simulink model "uz_pmsm_model_9ph"  (R2021b)
settings: Solver=FixedStepAuto  StartTime=0.0  StopTime=0.8  RelTol=1e-3
PreLoadFcn:
  | uz_pmsm_model_9ph_init_parameter
values from neighbouring files (symbols this model uses):
  c = 2/9*cat(1,tl1,tl2,tl3,tl4,tl5,tl6,tl7,tl8,tl9)    [uz_pmsm_model_9ph_init_parameter.m]
  friction_coefficient = 0.001    [uz_pmsm_model_9ph_init_parameter.m]
  inertia = 0.001    [uz_pmsm_model_9ph_init_parameter.m]
  k_i_d = 50    [uz_pmsm_model_9ph_init_parameter.m]
  k_i_q = 50    [uz_pmsm_model_9ph_init_parameter.m]
  k_p_d = 0.5    [uz_pmsm_model_9ph_init_parameter.m]
  k_p_q = 0.5    [uz_pmsm_model_9ph_init_parameter.m]
  L_d = 0.0023    [uz_pmsm_model_9ph_init_parameter.m]
  L_o1 = L_d/3    (= 0.000766666666667)    [uz_pmsm_model_9ph_init_parameter.m]
  L_o2 = L_d/3    (= 0.000766666666667)    [uz_pmsm_model_9ph_init_parameter.m]
  L_q = 0.0046    [uz_pmsm_model_9ph_init_parameter.m]
  L_x1 = L_d/3    (= 0.000766666666667)    [uz_pmsm_model_9ph_init_parameter.m]
  L_x2 = L_d/3    (= 0.000766666666667)    [uz_pmsm_model_9ph_init_parameter.m]
  L_y1 = L_d/3    (= 0.000766666666667)    [uz_pmsm_model_9ph_init_parameter.m]
  L_y2 = L_d/3    (= 0.000766666666667)    [uz_pmsm_model_9ph_init_parameter.m]
  L_zero = L_d/3    (= 0.000766666666667)    [uz_pmsm_model_9ph_init_parameter.m]
  polepair = 3    [uz_pmsm_model_9ph_init_parameter.m]
  psi_pm = 0.1028    [uz_pmsm_model_9ph_init_parameter.m]
  R_1 = 0.066    [uz_pmsm_model_9ph_init_parameter.m]
  static_friction_torque = 0.001    [uz_pmsm_model_9ph_init_parameter.m]
  ts = 2/1e6    (= 2e-06)    [uz_pmsm_model_9ph_init_parameter.m]
undefined symbols (not defined in the file or in its folder): Kpd, Tnd
libraries: slpidlib x2, simulink x2, spsAlphaBetaZerotodq0Lib x1, pid_lib x1, spsdq0toAlphaBetaZeroLib x1
(part 1 of 2)
settings Model: DataTypeOverride=Off  Creator=ts  LastModifiedBy=ts
settings SolverCC: AlgebraicLoopSolver=TrustRegion  AutoInsertRateTranBlk=on
settings DataIOCC: LimitDataPoints=on  SaveOutput=off  SaveTime=off
settings OptimizationCC: BlockReduction=off  ConditionallyExecuteInputs=off  DefaultParameterBehavior=Inlined  LifeSpan=inf
settings DebuggingCC: AlgebraicLoopMsg=error  SingleTaskRateTransMsg=error  AllowSymbolicDim=off  StrictBusMsg=ErrorOnBusTreatedAsVector  SFUnexpectedBacktrackingDiag=warning  SFNoUnconditionalDefaultTransitionDiag=warning  SFExecutionAtInitializationDiag=none  SFMachineParentedDataDiag=warning  ArithmeticOperatorsInVariantConditions=warning
settings HardwareCC: ProdBitPerPointer=32  ProdBitPerSizeT=32  ProdBitPerPtrDiffT=32  ProdLargestAtomicFloat=None  ProdIntDivRoundTo=Undefined  ProdEndianess=Unspecified  ProdWordSize=32  ProdHWDeviceType=ASIC/FPGA->ASIC/FPGA  ProdEqTarget=off
settings SFSimCC: SimUseLocalCustomCode=off  CustomCodeUndefinedFunction=UseInterfaceOnly
settings RTWCC: RTWUseLocalCustomCode=off
settings CodeAppCC: StateflowObjectComments=on
settings GRTTargetCC: TargetLangStandard=C89/C90 (ANSI)
settings ConfigComp: CovScope=ReferencedModels  CovMetricSettings=dw  CovSaveCumulativeToWorkspaceVar=on  CovSaveSingleToWorkspaceVar=on  CovExternalEMLEnable=off  CovSFcnEnable=off

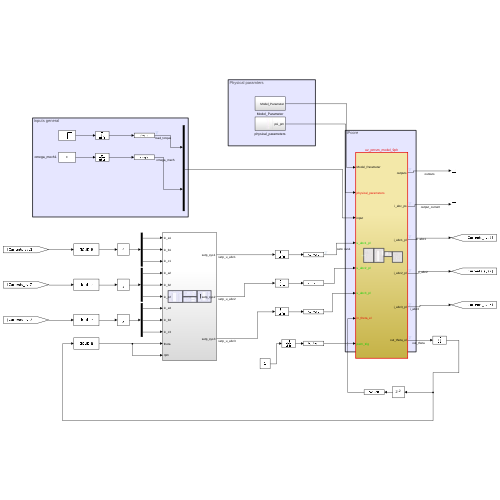
[thumbnail: Simulink's stored preview of the top-level diagram]
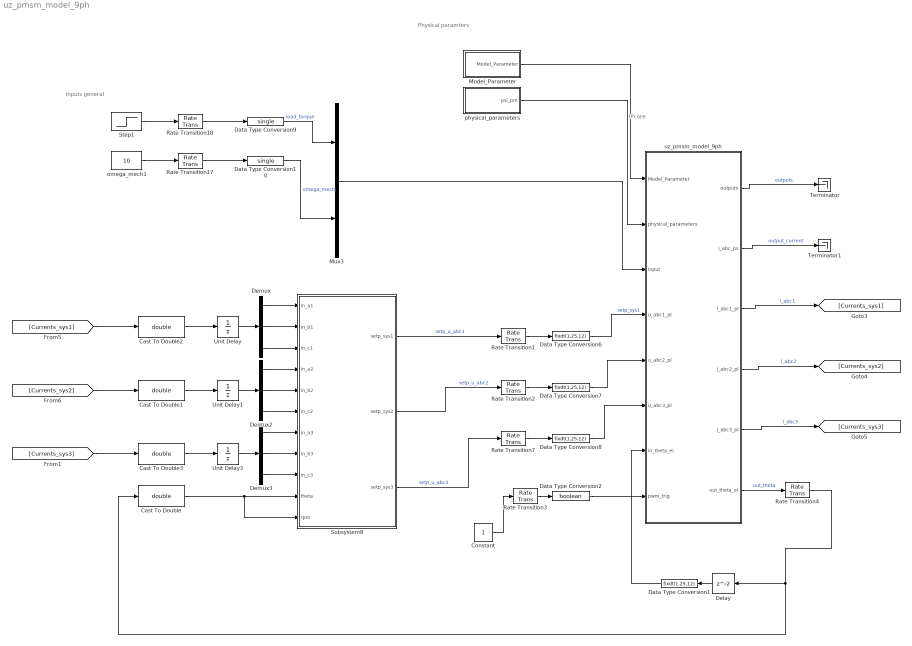
== system uz_pmsm_model_9ph ==
  note: IPcore
  note: Physical paramters
  note: Inputs general
  Cast To Double{,1..3} (4 alike) : DataTypeConversion  OutDataTypeStr=double
  Constant : Constant
  Data Type Conversion{1,6..8} (4 alike) : DataTypeConversion  OutDataTypeStr=fixdt(1,25,12)  RndMeth=Nearest
  Data Type Conversion10 : DataTypeConversion  OutDataTypeStr=single  RndMeth=Nearest
  Data Type Conversion2 : DataTypeConversion  OutDataTypeStr=boolean  RndMeth=Nearest
  Data Type Conversion9 : DataTypeConversion  OutDataTypeStr=single  RndMeth=Nearest
  Delay : Delay
  Demux : Demux  Outputs=3
  Demux2 : Demux  Outputs=3
  Demux3 : Demux  Outputs=3
  Model_Parameter : Subsystem
  Mux3 : Mux  Inputs=2
  Rate Transition{1..4,7,17..18} (7 alike) : RateTransition  OutPortSampleTime=ts
  Step1 : Step  Time=0.25  After=20  SampleTime=0
  Subsystem8 : Subsystem
  Terminator : Terminator
  Terminator1 : Terminator
  Unit Delay : UnitDelay  SampleTime=-1  HasFrameUpgradeWarning=on
  Unit Delay1 : UnitDelay  SampleTime=-1  HasFrameUpgradeWarning=on
  Unit Delay3 : UnitDelay  SampleTime=-1  HasFrameUpgradeWarning=on
  omega_mech1 : Constant  Value=10
  physical_parameters : Subsystem
  uz_pmsm_model_9ph : Subsystem  TreatAsAtomicUnit=on
  wires:
  physical_parameters/1(psi_pm) -> uz_pmsm_model_9ph/2(physical_parameters)
  uz_pmsm_model_9ph/1(outputs) -> Terminator/1  "outputs"
  Model_Parameter/1(Model_Parameter) -> uz_pmsm_model_9ph/1(Model_Parameter)
  omega_mech1/1 -> Rate Transition17/1
  Rate Transition18/1 -> Data Type Conversion9/1
  Step1/1 -> Rate Transition18/1
  Data Type Conversion10/1 -> Mux3/2  "omega_mech"
  Rate Transition17/1 -> Data Type Conversion10/1
  Data Type Conversion9/1 -> Mux3/1  "load_torque"
  Mux3/1 -> uz_pmsm_model_9ph/3(input)
  Data Type Conversion1/1 -> uz_pmsm_model_9ph/7(in_theta_el)
  uz_pmsm_model_9ph/2(i_abc_ps) -> Terminator1/1  "output_current"
  uz_pmsm_model_9ph/3(i_abc1_pl) -> [Currents_sys1]  "i_abc1"
  uz_pmsm_model_9ph/5(i_abc3_pl) -> [Currents_sys3]  "i_abc3"
  uz_pmsm_model_9ph/4(i_abc2_pl) -> [Currents_sys2]  "i_abc2"
  uz_pmsm_model_9ph/6(out_theta_el) -> Rate Transition4/1  "out_theta"
  Delay/1 -> Data Type Conversion1/1
  Subsystem8/1(setp_sys1) -> Rate Transition1/1  "setp_u_abc1"
  Data Type Conversion6/1 -> uz_pmsm_model_9ph/4(u_abc1_pl)  "setp_sys1"
  Subsystem8/2(setp_sys2) -> Rate Transition2/1  "setp_u_abc2"
  Subsystem8/3(setp_sys3) -> Rate Transition7/1  "setp_u_abc3"
  Data Type Conversion8/1 -> uz_pmsm_model_9ph/6(u_abc3_pl)
  Data Type Conversion7/1 -> uz_pmsm_model_9ph/5(u_abc2_pl)
  Unit Delay3/1 -> Demux3/1
  Demux/2 -> Subsystem8/2(in_b1)
  Demux2/1 -> Subsystem8/4(in_a2)
  Demux3/2 -> Subsystem8/8(in_b3)
  Unit Delay1/1 -> Demux2/1
  Demux/3 -> Subsystem8/3(in_c1)
  [Currents_sys1] -> Cast To Double2/1
  [Currents_sys2] -> Cast To Double1/1
  Demux3/3 -> Subsystem8/9(in_c3)
  Unit Delay/1 -> Demux/1
  [Currents_sys3] -> Cast To Double3/1
  Demux3/1 -> Subsystem8/7(in_a3)
  Demux/1 -> Subsystem8/1(in_a1)
  Demux2/2 -> Subsystem8/5(in_b2)
  Demux2/3 -> Subsystem8/6(in_c2)
  Cast To Double/1 -> Subsystem8/11(rpm), Subsystem8/10(theta)
  Cast To Double1/1 -> Unit Delay1/1
  Cast To Double2/1 -> Unit Delay/1
  Cast To Double3/1 -> Unit Delay3/1
  Rate Transition1/1 -> Data Type Conversion6/1
  Rate Transition2/1 -> Data Type Conversion7/1
  Rate Transition7/1 -> Data Type Conversion8/1
  Data Type Conversion2/1 -> uz_pmsm_model_9ph/8(pwm_trig)
  Rate Transition3/1 -> Data Type Conversion2/1
  Constant/1 -> Rate Transition3/1
  Rate Transition4/1 -> Delay/1, Cast To Double/1

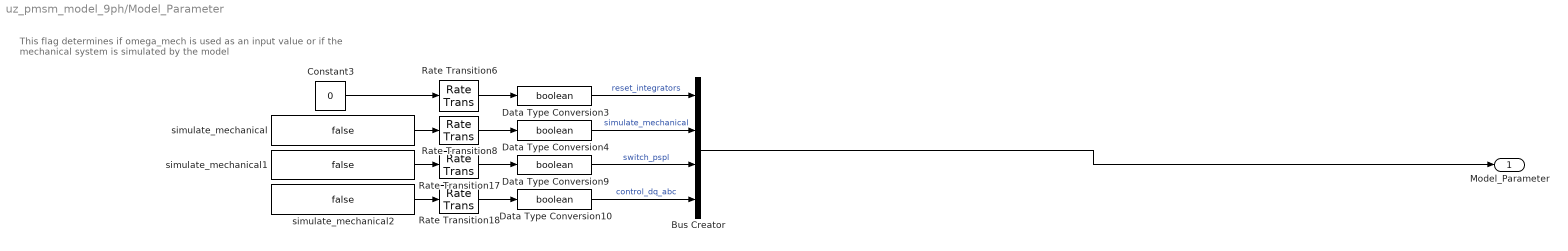
== system uz_pmsm_model_9ph/Model_Parameter ==
  note: This flag determines if omega_mech is used as an input value or
      | if the mechanical system is simulated by the model
  Bus Creator : BusCreator  Inputs=4
  Constant3 : Constant  Value=0
  Data Type Conversion{3..4,9..10} (4 alike) : DataTypeConversion  OutDataTypeStr=boolean
  Rate Transition{6,8,17..18} (4 alike) : RateTransition  OutPortSampleTime=ts
  simulate_mechanical : Constant  Value=false
  simulate_mechanical1 : Constant  Value=false
  simulate_mechanical2 : Constant  Value=false
  Model_Parameter : Outport
  wires:
  simulate_mechanical2/1 -> Rate Transition18/1
  simulate_mechanical/1 -> Rate Transition8/1
  Rate Transition8/1 -> Data Type Conversion4/1
  Rate Transition6/1 -> Data Type Conversion3/1
  Constant3/1 -> Rate Transition6/1
  simulate_mechanical1/1 -> Rate Transition17/1
  Rate Transition17/1 -> Data Type Conversion9/1
  Rate Transition18/1 -> Data Type Conversion10/1
  Data Type Conversion10/1 -> Bus Creator/4  "control_dq_abc"
  Data Type Conversion9/1 -> Bus Creator/3  "switch_pspl"
  Data Type Conversion4/1 -> Bus Creator/2  "simulate_mechanical"
  Bus Creator/1 -> Model_Parameter/1
  Data Type Conversion3/1 -> Bus Creator/1  "reset_integrators"

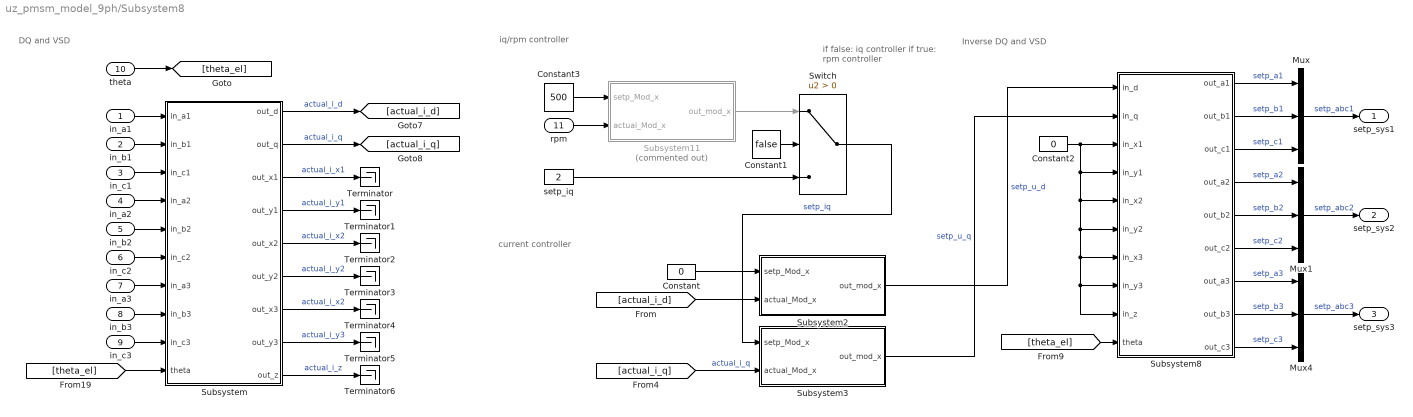
== system uz_pmsm_model_9ph/Subsystem8 ==
  note: DQ and VSD
  note: current controller
  note: iq/rpm controller
  note: if false: iq controller
      | if true: rpm controller
  note: Inverse DQ and VSD
  in_a1 : Inport
  in_b1 : Inport  Port=2
  in_c1 : Inport  Port=3
  in_a2 : Inport  Port=4
  in_b2 : Inport  Port=5
  in_c2 : Inport  Port=6
  in_a3 : Inport  Port=7
  in_b3 : Inport  Port=8
  in_c3 : Inport  Port=9
  theta : Inport  Port=10
  rpm : Inport  Port=11
  Constant : Constant  Value=0
  Constant1 : Constant  Value=false
  Constant2 : Constant  Value=0
  Constant3 : Constant  Value=500
  Mux : Mux  Inputs=3
  Mux1 : Mux  Inputs=3
  Mux4 : Mux  Inputs=3
  Subsystem : Subsystem
  Subsystem11 : Subsystem  Commented=on
  Subsystem2 : Subsystem
  Subsystem3 : Subsystem
  Subsystem8 : Subsystem
  Switch : Switch  Criteria=u2 > Threshold
  Terminator{,1..6} (7 alike) : Terminator
  setp_iq : Constant  Value=2
  setp_sys1 : Outport
  setp_sys2 : Outport  Port=2
  setp_sys3 : Outport  Port=3
  wires:
  Subsystem/4(out_y1) -> Terminator1/1  "actual_i_y1"
  Subsystem8/1(out_a1) -> Mux/1  "setp_a1"
  in_b1/1 -> Subsystem/2(in_b1)
  [theta_el] -> Subsystem8/10(theta)
  Subsystem8/2(out_b1) -> Mux/2  "setp_b1"
  Subsystem8/3(out_c1) -> Mux/3  "setp_c1"
  Subsystem/3(out_x1) -> Terminator/1  "actual_i_x1"
  in_c1/1 -> Subsystem/3(in_c1)
  [actual_i_d] -> Subsystem2/2(actual_Mod_x)
  Constant/1 -> Subsystem2/1(setp_Mod_x)
  Subsystem/6(out_y2) -> Terminator3/1  "actual_i_y2"
  Subsystem/5(out_x2) -> Terminator2/1  "actual_i_x2"
  in_a1/1 -> Subsystem/1(in_a1)
  [actual_i_q] -> Subsystem3/2(actual_Mod_x)  "actual_i_q"
  in_b2/1 -> Subsystem/5(in_b2)
  in_a2/1 -> Subsystem/4(in_a2)
  in_c2/1 -> Subsystem/6(in_c2)
  theta/1 -> [theta_el]
  Mux/1 -> setp_sys1/1  "setp_abc1"
  Subsystem/8(out_y3) -> Terminator5/1  "actual_i_y3"
  Subsystem/7(out_x3) -> Terminator4/1  "actual_i_x2"
  Subsystem/9(out_z) -> Terminator6/1  "actual_i_z"
  in_c3/1 -> Subsystem/9(in_c3)
  in_b3/1 -> Subsystem/8(in_b3)
  in_a3/1 -> Subsystem/7(in_a3)
  Mux1/1 -> setp_sys2/1  "setp_abc2"
  Subsystem8/6(out_c2) -> Mux1/3  "setp_c2"
  Subsystem8/5(out_b2) -> Mux1/2  "setp_b2"
  Subsystem8/4(out_a2) -> Mux1/1  "setp_a2"
  Mux4/1 -> setp_sys3/1  "setp_abc3"
  Subsystem8/7(out_a3) -> Mux4/1  "setp_a3"
  Subsystem8/8(out_b3) -> Mux4/2  "setp_b3"
  Subsystem8/9(out_c3) -> Mux4/3  "setp_c3"
  rpm/1 -> Subsystem11/2(actual_Mod_x)
  Subsystem/1(out_d) -> [actual_i_d]  "actual_i_d"
  Subsystem/2(out_q) -> [actual_i_q]  "actual_i_q"
  [theta_el] -> Subsystem/10(theta)
  Constant2/1 -> Subsystem8/3(in_x1), Subsystem8/8(in_y3), Subsystem8/9(in_z), Subsystem8/7(in_x3), Subsystem8/6(in_y2), Subsystem8/5(in_x2), Subsystem8/4(in_y1)
  Subsystem11/1(out_mod_x) -> Switch/1
  Switch/1 -> Subsystem3/1(setp_Mod_x)  "setp_iq"
  Constant1/1 -> Switch/2
  setp_iq/1 -> Switch/3
  Constant3/1 -> Subsystem11/1(setp_Mod_x)
  Subsystem3/1(out_mod_x) -> Subsystem8/2(in_q)  "setp_u_q"
  Subsystem2/1(out_mod_x) -> Subsystem8/1(in_d)  "setp_u_d"

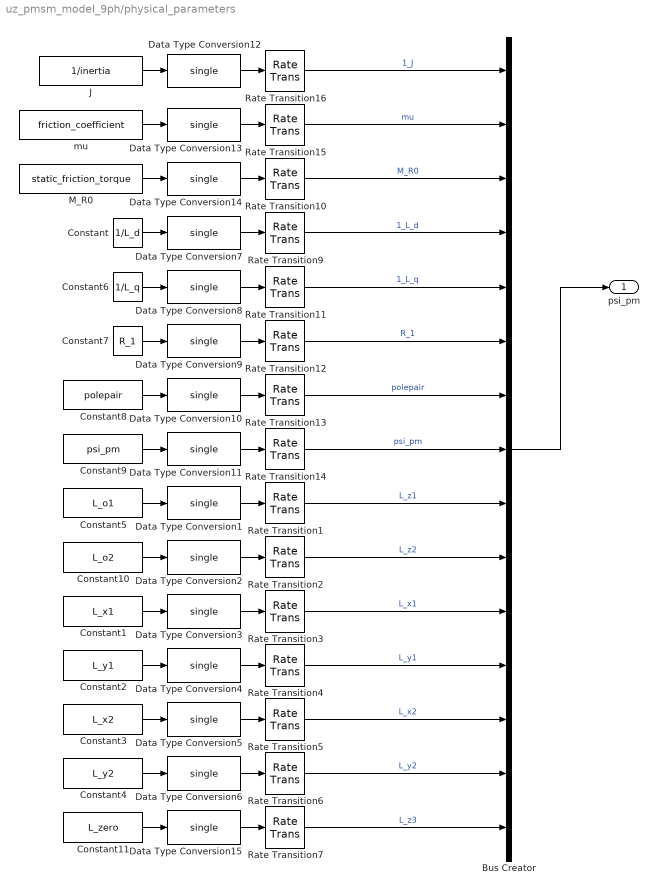
== system uz_pmsm_model_9ph/physical_parameters ==
  Bus Creator : BusCreator  Inputs=15
  Constant : Constant  Value=1/L_d
  Constant1 : Constant  Value=L_x1
  Constant10 : Constant  Value=L_o2
  Constant11 : Constant  Value=L_zero
  Constant2 : Constant  Value=L_y1
  Constant3 : Constant  Value=L_x2
  Constant4 : Constant  Value=L_y2
  Constant5 : Constant  Value=L_o1
  Constant6 : Constant  Value=1/L_q
  Constant7 : Constant  Value=R_1
  Constant8 : Constant  Value=polepair
  Constant9 : Constant  Value=psi_pm
  Data Type Conversion{1..15} (15 alike) : DataTypeConversion  OutDataTypeStr=single
  J : Constant  Value=1/inertia
  M_R0 : Constant  Value=static_friction_torque
  Rate Transition{1..7,9..16} (15 alike) : RateTransition  OutPortSampleTime=ts
  mu : Constant  Value=friction_coefficient
  psi_pm : Outport
  wires:
  Data Type Conversion12/1 -> Rate Transition16/1
  Data Type Conversion7/1 -> Rate Transition9/1
  Rate Transition10/1 -> Bus Creator/3  "M_R0"
  Rate Transition14/1 -> Bus Creator/8  "psi_pm"
  Data Type Conversion14/1 -> Rate Transition10/1
  Rate Transition12/1 -> Bus Creator/6  "R_1"
  Rate Transition16/1 -> Bus Creator/1  "1_J"
  Rate Transition13/1 -> Bus Creator/7  "polepair"
  Bus Creator/1 -> psi_pm/1
  Data Type Conversion11/1 -> Rate Transition14/1
  Constant8/1 -> Data Type Conversion10/1
  Data Type Conversion9/1 -> Rate Transition12/1
  Rate Transition15/1 -> Bus Creator/2  "mu"
  Constant6/1 -> Data Type Conversion8/1
  Rate Transition9/1 -> Bus Creator/4  "1_L_d"
  J/1 -> Data Type Conversion12/1
  Data Type Conversion8/1 -> Rate Transition11/1
  Data Type Conversion10/1 -> Rate Transition13/1
  mu/1 -> Data Type Conversion13/1
  M_R0/1 -> Data Type Conversion14/1
  Rate Transition11/1 -> Bus Creator/5  "1_L_q"
  Data Type Conversion13/1 -> Rate Transition15/1
  Constant7/1 -> Data Type Conversion9/1
  Constant9/1 -> Data Type Conversion11/1
  Constant/1 -> Data Type Conversion7/1
  Data Type Conversion1/1 -> Rate Transition1/1
  Data Type Conversion2/1 -> Rate Transition2/1
  Data Type Conversion3/1 -> Rate Transition3/1
  Data Type Conversion4/1 -> Rate Transition4/1
  Data Type Conversion5/1 -> Rate Transition5/1
  Data Type Conversion6/1 -> Rate Transition6/1
  Constant11/1 -> Data Type Conversion15/1
  Data Type Conversion15/1 -> Rate Transition7/1
  Rate Transition1/1 -> Bus Creator/9  "L_z1"
  Rate Transition7/1 -> Bus Creator/15  "L_z3"
  Rate Transition6/1 -> Bus Creator/14  "L_y2"
  Rate Transition5/1 -> Bus Creator/13  "L_x2"
  Rate Transition4/1 -> Bus Creator/12  "L_y1"
  Rate Transition3/1 -> Bus Creator/11  "L_x1"
  Rate Transition2/1 -> Bus Creator/10  "L_z2"
  Constant4/1 -> Data Type Conversion6/1
  Constant3/1 -> Data Type Conversion5/1
  Constant2/1 -> Data Type Conversion4/1
  Constant1/1 -> Data Type Conversion3/1
  Constant5/1 -> Data Type Conversion1/1
  Constant10/1 -> Data Type Conversion2/1

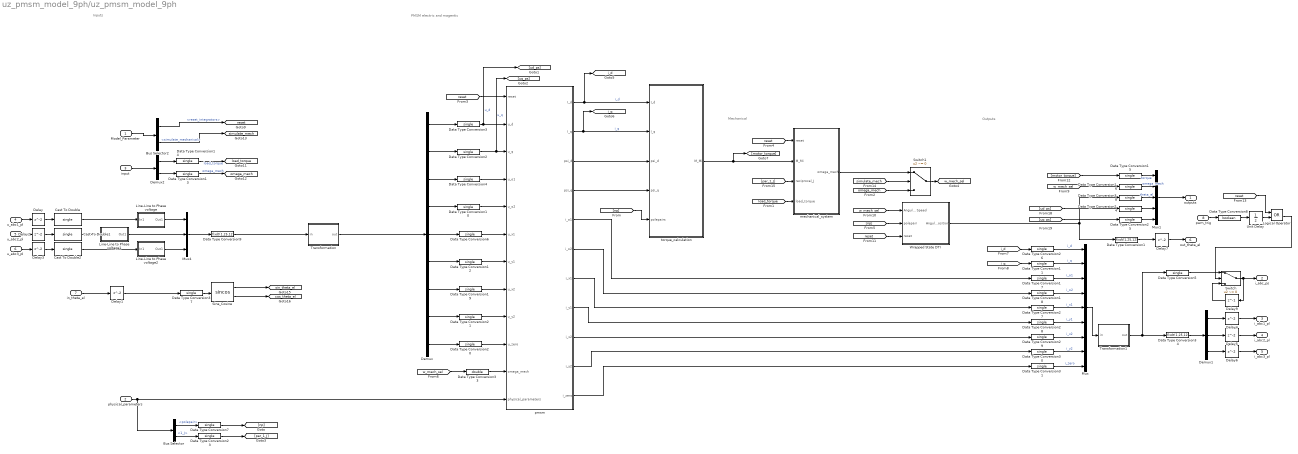
== system uz_pmsm_model_9ph/uz_pmsm_model_9ph ==
  note: PMSM electric and magentic
  note: Mechanical
  note: Outputs
  note: Inputs
  Model_Parameter : Inport
  physical_parameters : Inport  Port=2
  input : Inport  Port=3
  u_abc1_pl : Inport  Port=4
  u_abc2_pl : Inport  Port=5
  u_abc3_pl : Inport  Port=6
  in_theta_el : Inport  Port=7
  pwm_trig : Inport  Port=8
  Bus Selector : BusSelector  OutputSignals=polepair,1_J
  Bus Selector2 : BusSelector  OutputSignals=reset_integrators,simulate_mechanical
  Cast To Double : DataTypeConversion  OutDataTypeStr=single
  Cast To Double1 : DataTypeConversion  OutDataTypeStr=single
  Cast To Double2 : DataTypeConversion  OutDataTypeStr=single
  Data Type Conversion1 : DataTypeConversion  OutDataTypeStr=fixdt(1,25,12)  RndMeth=Nearest
  Data Type Conversion{2..7,10..21,23..31,37..38} (29 alike) : DataTypeConversion  OutDataTypeStr=single  RndMeth=Nearest
  Data Type Conversion33 : DataTypeConversion  OutDataTypeStr=double  RndMeth=Nearest
  Data Type Conversion34 : DataTypeConversion  OutDataTypeStr=fixdt(1,25,12)  RndMeth=Nearest
  Data Type Conversion8 : DataTypeConversion  OutDataTypeStr=boolean  RndMeth=Nearest
  Data Type Conversion9 : DataTypeConversion  OutDataTypeStr=fixdt(1,25,12)  RndMeth=Nearest
  Delay{,1..7} (8 alike) : Delay
  Delay9 : Delay  DelayLength=1
  Demux : Demux  Outputs=9
  Demux1 : Demux  Outputs=3
  Demux2 : Demux  Outputs=2
  Line-Line to Phase voltage : Subsystem
  Line-Line to Phase voltage1 : Subsystem
  Line-Line to Phase voltage2 : Subsystem
  Logical Operator : Logic  Operator=OR  AllPortsSameDT=off  OutDataTypeStr=boolean
  Mux : Mux  Inputs=9
  Mux1 : Mux  Inputs=5
  Mux4 : Mux  Inputs=3
  Sine_Cosine : Trigonometry  Operator=sincos
  Switch : Switch  Criteria=u2 ~= 0
  Switch1 : Switch  Criteria=u2 ~= 0
  Transformation : Subsystem
  Transformation1 : Subsystem
  Unit Delay : UnitDelay  SampleTime=-1  HasFrameUpgradeWarning=on
  Wrapped State DTI : Subsystem
  mechanical_system : Subsystem
  pmsm : Subsystem
  torque_calculation : Subsystem
  outputs : Outport
  i_abc_ps : Outport  Port=2
  i_abc1_pl : Outport  Port=3
  i_abc2_pl : Outport  Port=4
  i_abc3_pl : Outport  Port=5
  out_theta_el : Outport  Port=6
  tag scope: cos_theta_el=global, i_d=global, i_q=global, load_torque=global, omega_mech=global, reset=global, simulate_mech=global, sin_theta_el=global, w_mech_sel=global
  wires:
  pmsm/3(psi_d) -> torque_calculation/3(psi_d)
  pmsm/4(psi_q) -> torque_calculation/4(psi_q)
  Data Type Conversion3/1 -> [ud_ps], pmsm/2(u_d)  "u_d"
  [simulate_mech] -> Switch1/2
  torque_calculation/1(M_Mi) -> [motor_torque], mechanical_system/2(M_Mi)
  physical_parameters/1 -> pmsm/12(physical_parameters), Bus Selector/1
  Data Type Conversion2/1 -> [uq_ps], pmsm/3(u_q)  "u_q"
  mechanical_system/1(omega_mech) -> Switch1/1
  pmsm/2(I_q) -> [i_q], torque_calculation/2(I_q)  "i_q"
  pmsm/1(I_d) -> [i_d], torque_calculation/1(I_d)  "i_d"
  Data Type Conversion16/1 -> Mux1/2  "omega_mech"
  Data Type Conversion15/1 -> Mux1/1  "torque"
  Data Type Conversion11/1 -> Mux/2  "i_q"
  Demux/1 -> Data Type Conversion3/1
  Demux/2 -> Data Type Conversion2/1
  [np] -> torque_calculation/5(polepairs)
  [load_torque] -> mechanical_system/4(load_torque)
  [omega_mech] -> Switch1/3
  Demux/3 -> Data Type Conversion4/1
  Demux/4 -> Data Type Conversion10/1
  Demux/5 -> Data Type Conversion6/1
  Demux/6 -> Data Type Conversion12/1
  Demux/7 -> Data Type Conversion19/1
  Demux/8 -> Data Type Conversion21/1
  Demux/9 -> Data Type Conversion20/1
  Data Type Conversion4/1 -> pmsm/4(u_o1)
  Data Type Conversion10/1 -> pmsm/5(u_o2)
  Data Type Conversion6/1 -> pmsm/6(u_x1)
  Data Type Conversion12/1 -> pmsm/7(u_y1)
  Data Type Conversion19/1 -> pmsm/8(u_x2)
  Data Type Conversion20/1 -> pmsm/10(u_zero)
  Data Type Conversion17/1 -> Mux/3  "i_o1"
  Data Type Conversion18/1 -> Mux/4  "i_o2"
  pmsm/5(i_o1) -> Data Type Conversion17/1
  Data Type Conversion27/1 -> Mux/5  "i_x1"
  Data Type Conversion28/1 -> Mux/6  "i_y1"
  Data Type Conversion29/1 -> Mux/7  "i_x2"
  Data Type Conversion30/1 -> Mux/8  "i_y2"
  Data Type Conversion31/1 -> Mux/9  "i_zero"
  [reset] -> pmsm/1(reset)
  [reset] -> mechanical_system/1(reset)
  Data Type Conversion21/1 -> pmsm/9(u_y2)
  pmsm/6(i_o2) -> Data Type Conversion18/1
  pmsm/7(i_x1) -> Data Type Conversion27/1
  pmsm/8(i_y1) -> Data Type Conversion28/1
  pmsm/9(i_x2) -> Data Type Conversion29/1
  pmsm/10(i_y2) -> Data Type Conversion30/1
  pmsm/11(i_zero) -> Data Type Conversion31/1
  Data Type Conversion38/1 -> Mux1/3  "theta_el"
  [i_q] -> Data Type Conversion11/1
  [i_d] -> Data Type Conversion26/1
  [w_mech_sel] -> Data Type Conversion16/1
  [np] -> Wrapped State DTI/2(polepair)
  [reset] -> Wrapped State DTI/3(reset)
  [motor_torque] -> Data Type Conversion15/1
  Bus Selector/1 -> Data Type Conversion7/1  "<polepair>"
  Data Type Conversion7/1 -> [np]
  [par_1_J] -> mechanical_system/3(reciprocal_J)
  Data Type Conversion14/1 -> [load_torque]  "load_torque"
  u_abc1_pl/1 -> Delay/1
  Data Type Conversion9/1 -> Transformation/1(in)
  u_abc2_pl/1 -> Delay2/1
  u_abc3_pl/1 -> Delay3/1
  Demux2/2 -> Data Type Conversion13/1
  Data Type Conversion13/1 -> [omega_mech]  "omega_mech"
  input/1 -> Demux2/1
  Mux4/1 -> Data Type Conversion9/1
  Model_Parameter/1 -> Bus Selector2/1
  Demux2/1 -> Data Type Conversion14/1
  Bus Selector2/1 -> [reset]  "<reset_integrators>"
  Bus Selector2/2 -> [simulate_mech]  "<simulate_mechanical>"
  Data Type Conversion26/1 -> Mux/1  "i_d"
  Mux1/1 -> outputs/1
  Mux/1 -> Transformation1/1(in)
  Transformation1/1(out) -> Data Type Conversion34/1, Data Type Conversion5/1
  Data Type Conversion34/1 -> Demux1/1
  Switch1/1 -> [w_mech_sel]
  Demux1/1 -> Delay4/1
  Demux1/3 -> Delay6/1
  Demux1/2 -> Delay5/1
  Wrapped State DTI/1(Angular Position) -> Data Type Conversion38/1, Data Type Conversion1/1
  [w_mech_sel] -> Wrapped State DTI/1(Angular Speed)
  in_theta_el/1 -> Delay1/1
  Data Type Conversion1/1 -> Delay7/1
  [w_mech_sel] -> Data Type Conversion33/1
  Data Type Conversion23/1 -> [par_1_J]
  Bus Selector/2 -> Data Type Conversion23/1  "<1_J>"
  Delay4/1 -> i_abc1_pl/1
  Delay5/1 -> i_abc2_pl/1
  Delay6/1 -> i_abc3_pl/1
  Delay7/1 -> out_theta_el/1
  Transformation/1(out) -> Demux/1
  Data Type Conversion24/1 -> Mux1/4
  Data Type Conversion25/1 -> Mux1/5
  [ud_ps] -> Data Type Conversion24/1
  [uq_ps] -> Data Type Conversion25/1
  Data Type Conversion33/1 -> pmsm/11(omega_mech)
  Data Type Conversion37/1 -> Sine_Cosine/1
  Delay1/1 -> Data Type Conversion37/1
  Delay/1 -> Cast To Double/1
  Cast To Double/1 -> Line-Line to Phase voltage/1(In1)
  Line-Line to Phase voltage/1(Out1) -> Mux4/1
  Line-Line to Phase voltage1/1(Out1) -> Mux4/2
  Cast To Double1/1 -> Line-Line to Phase voltage1/1(In1)
  Cast To Double2/1 -> Line-Line to Phase voltage2/1(In1)
  Line-Line to Phase voltage2/1(Out1) -> Mux4/3
  Delay2/1 -> Cast To Double1/1
  Delay3/1 -> Cast To Double2/1
  Sine_Cosine/1 -> [sin_theta_el]
  Sine_Cosine/2 -> [cos_theta_el]
  Data Type Conversion5/1 -> Switch/1
  Delay9/1 -> Switch/3
  Switch/1 -> i_abc_ps/1, Delay9/1
  pwm_trig/1 -> Data Type Conversion8/1
  Data Type Conversion8/1 -> Unit Delay/1
  Unit Delay/1 -> Logical Operator/2
  Logical Operator/1 -> Switch/2
  [reset] -> Logical Operator/1

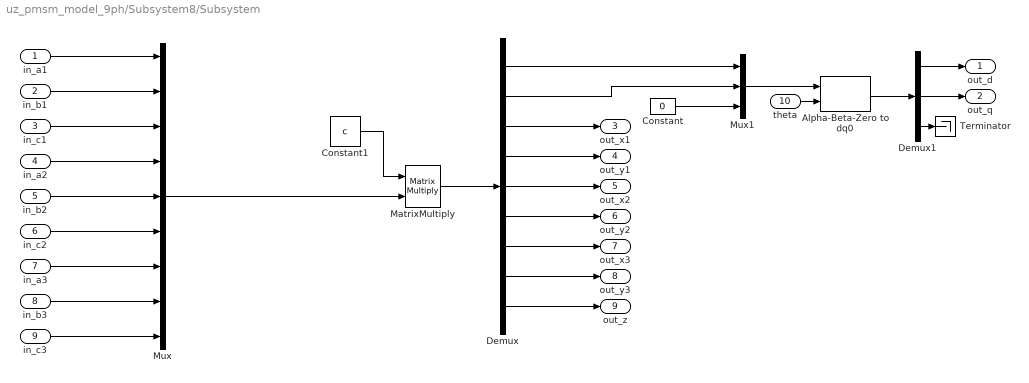
== system uz_pmsm_model_9ph/Subsystem8/Subsystem ==
  in_a1 : Inport
  in_b1 : Inport  Port=2
  in_c1 : Inport  Port=3
  in_a2 : Inport  Port=4
  in_b2 : Inport  Port=5
  in_c2 : Inport  Port=6
  in_a3 : Inport  Port=7
  in_b3 : Inport  Port=8
  in_c3 : Inport  Port=9
  theta : Inport  Port=10
  Alpha-Beta-Zero to dq0 : spsAlphaBetaZerotodq0Lib/Alpha-Beta-Zero to dq0  Alignment=90 degrees behind phase A axis
      settings: SourceProductBaseCode=PS
  Constant : Constant  Value=0
  Constant1 : Constant  Value=c
  Demux : Demux  Outputs=9
  Demux1 : Demux  Outputs=3
  MatrixMultiply : Product  Multiplication=Matrix(*)
  Mux : Mux  Inputs=9
  Mux1 : Mux  Inputs=3
  Terminator : Terminator
  out_d : Outport
  out_q : Outport  Port=2
  out_x1 : Outport  Port=3
  out_y1 : Outport  Port=4
  out_x2 : Outport  Port=5
  out_y2 : Outport  Port=6
  out_x3 : Outport  Port=7
  out_y3 : Outport  Port=8
  out_z : Outport  Port=9
  wires:
  Demux/6 -> out_y2/1
  Demux/4 -> out_y1/1
  in_a1/1 -> Mux/1
  Demux/5 -> out_x2/1
  MatrixMultiply/1 -> Demux/1
  Demux/3 -> out_x1/1
  in_c3/1 -> Mux/9
  Demux/7 -> out_x3/1
  Demux/8 -> out_y3/1
  Demux/9 -> out_z/1
  theta/1 -> Alpha-Beta-Zero to dq0/2
  Demux1/3 -> Terminator/1
  Demux/1 -> Mux1/1
  Mux1/1 -> Alpha-Beta-Zero to dq0/1
  Demux/2 -> Mux1/2
  Demux1/1 -> out_d/1
  Demux1/2 -> out_q/1
  Constant/1 -> Mux1/3
  Alpha-Beta-Zero to dq0/1 -> Demux1/1
  Constant1/1 -> MatrixMultiply/1
  Mux/1 -> MatrixMultiply/2
  in_b1/1 -> Mux/2
  in_c1/1 -> Mux/3
  in_a2/1 -> Mux/4
  in_b2/1 -> Mux/5
  in_c2/1 -> Mux/6
  in_a3/1 -> Mux/7
  in_b3/1 -> Mux/8

== system uz_pmsm_model_9ph/Subsystem8/Subsystem11 ==
  setp_Mod_x : Inport
  actual_Mod_x : Inport  Port=2
  Add : Sum  Inputs=+-
  Data Type Conversion8 : DataTypeConversion  OutDataTypeStr=double
  PID Controller2 : pid_lib/PID Controller  Controller=PI  Form=Ideal  TimeDomain=Continuous-time  UseExternalTs=off  SampleTime=-1  IntegratorMethod=Forward Euler  FilterMethod=Forward Euler  ControllerParametersSource=internal  P=Kpd  I=1/Tnd  D=0  UseFilter=on  N=100  TunerSelectOption=Transfer Function Based (PID Tuner App)  InitialConditionSource=internal  InitialConditionForIntegrator=0  InitialConditionForFilter=0  DifferentiatorICPrevScaledInput=0  ExternalReset=none  TrackingMode=off  Kt=1  LimitOutput=on  SatLimitsSource=internal  UpperSaturationLimit=50  LowerSaturationLimit=-50  LinearizeAsGain=on  AntiWindupMode=clamping  Kb=1  POutMin=[]  POutMax=[]  IOutMin=[]  IOutMax=[]  DOutMin=[]  DOutMax=[]  NOutMin=[]  NOutMax=[]  SumOutMin=[]  SumOutMax=[]  SaturationOutMin=[]  SaturationOutMax=[]  PParamMin=[]  PParamMax=[]  IParamMin=[]  IParamMax=[]  DParamMin=[]  DParamMax=[]  NParamMin=[]  NParamMax=[]  KbParamMin=[]  KbParamMax=[]  KtParamMin=[]  KtParamMax=[]  KbOutMin=[]  KbOutMax=[]  KtOutMin=[]  KtOutMax=[]  IntegratorOutMin=[]  IntegratorOutMax=[]  FilterOutMin=[]  FilterOutMax=[]  SumI1OutMin=[]  SumI1OutMax=[]  SumI2OutMin=[]  SumI2OutMax=[]  SumI3OutMin=[]  SumI3OutMax=[]  SumI4OutMin=[]  SumI4OutMax=[]  SumDOutMin=[]  SumDOutMax=[]  DifferentiatorOutMin=[]  DifferentiatorOutMax=[]  FilterDiffOutCoefMin=[]  FilterDiffOutCoefMax=[]  ReciprocalOutMin=[]  ReciprocalOutMax=[]  SumDenOutMin=[]  SumDenOutMax=[]  SumNumOutMin=[]  SumNumOutMax=[]  DivideOutMin=[]  DivideOutMax=[]  UdiffTsProdOutMin=[]  UdiffTsProdOutMax=[]  NTsProdOutMin=[]  NTsProdOutMax=[]  UintegralTsProdOutMin=[]  UintegralTsProdOutMax=[]  UngainTsProdOutMin=[]  UngainTsProdOutMax=[]  IntegratorContinuousStateAttributes=''  IntegratorStateMustResolveToSignalObject=off  IntegratorRTWStateStorageClass=Auto  FilterContinuousStateAttributes=''  FilterStateMustResolveToSignalObject=off  FilterRTWStateStorageClass=Auto  ParallelPVariant=Passthrough  IdealPVariant=InternalParameters  IVariant=InternalParameters  DVariant=Disabled  IntegratorVariant=Continuous  SatVariant=Enabled  AWVariant=ContClampingIdeal  PCopyVariant=InternalParamsIdeal  TRVariant=Disabled  FdbkBlocksVariant=Forward  IdealPFdbkVariant=Disabled  SatFdbkVariant=Disabled  DerivativeFilterVariant=Disabled  NVariant=Disabled  NCopyVariant=Disabled_SignalSpec  FilterICVariant=Disabled  IntegratorICVariant=InternalICs  ExternalResetVariant=Disabled  TRSumVariant=Passthrough  SumFdbkVariant=Disabled  SumVariant=Sum_PI  TsampFilterVariant=InternalTs  TsampNgainVariant=Passthrough  TsampIntegralVariant=Passthrough  ExternalSaturationOutDataTypeStr=Inherit: Same as second input
  out_mod_x : Outport
  wires:
  Add/1 -> Data Type Conversion8/1
  actual_Mod_x/1 -> Add/2
  Data Type Conversion8/1 -> PID Controller2/1
  setp_Mod_x/1 -> Add/1
  PID Controller2/1 -> out_mod_x/1

== system uz_pmsm_model_9ph/Subsystem8/Subsystem2 ==
  setp_Mod_x : Inport
  actual_Mod_x : Inport  Port=2
  Add : Sum  Inputs=+-
  Data Type Conversion8 : DataTypeConversion  OutDataTypeStr=double
  PID Controller2 : slpidlib/PID Controller  Controller=PI  Form=Ideal  TimeDomain=Continuous-time  UseExternalTs=off  SampleTime=-1  IntegratorMethod=Forward Euler  FilterMethod=Forward Euler  ControllerParametersSource=internal  P=k_p_d  I=k_i_d  D=0  UseFilter=on  N=100  TunerSelectOption=Transfer Function Based (PID Tuner App)  InitialConditionSource=internal  InitialConditionForIntegrator=0  InitialConditionForFilter=0  DifferentiatorICPrevScaledInput=0  ExternalReset=none  TrackingMode=off  Kt=1  LimitOutput=on  SatLimitsSource=internal  UpperSaturationLimit=100  LowerSaturationLimit=-100  LinearizeAsGain=on  AntiWindupMode=clamping  Kb=1  POutMin=[]  POutMax=[]  IOutMin=[]  IOutMax=[]  DOutMin=[]  DOutMax=[]  NOutMin=[]  NOutMax=[]  SumOutMin=[]  SumOutMax=[]  SaturationOutMin=[]  SaturationOutMax=[]  PParamMin=[]  PParamMax=[]  IParamMin=[]  IParamMax=[]  DParamMin=[]  DParamMax=[]  NParamMin=[]  NParamMax=[]  KbParamMin=[]  KbParamMax=[]  KtParamMin=[]  KtParamMax=[]  KbOutMin=[]  KbOutMax=[]  KtOutMin=[]  KtOutMax=[]  IntegratorOutMin=[]  IntegratorOutMax=[]  FilterOutMin=[]  FilterOutMax=[]  SumI1OutMin=[]  SumI1OutMax=[]  SumI2OutMin=[]  SumI2OutMax=[]  SumI3OutMin=[]  SumI3OutMax=[]  SumI4OutMin=[]  SumI4OutMax=[]  SumDOutMin=[]  SumDOutMax=[]  DifferentiatorOutMin=[]  DifferentiatorOutMax=[]  FilterDiffOutCoefMin=[]  FilterDiffOutCoefMax=[]  ReciprocalOutMin=[]  ReciprocalOutMax=[]  SumDenOutMin=[]  SumDenOutMax=[]  SumNumOutMin=[]  SumNumOutMax=[]  DivideOutMin=[]  DivideOutMax=[]  UdiffTsProdOutMin=[]  UdiffTsProdOutMax=[]  NTsProdOutMin=[]  NTsProdOutMax=[]  UintegralTsProdOutMin=[]  UintegralTsProdOutMax=[]  UngainTsProdOutMin=[]  UngainTsProdOutMax=[]  IntegratorContinuousStateAttributes=''  IntegratorStateMustResolveToSignalObject=off  IntegratorRTWStateStorageClass=Auto  FilterContinuousStateAttributes=''  FilterStateMustResolveToSignalObject=off  FilterRTWStateStorageClass=Auto  ParallelPVariant=Passthrough  IdealPVariant=InternalParameters  IVariant=InternalParameters  DVariant=Disabled  IntegratorVariant=Continuous  SatVariant=Enabled  AWVariant=ContClampingIdeal  PCopyVariant=InternalParamsIdeal  TRVariant=Disabled  FdbkBlocksVariant=Forward  IdealPFdbkVariant=Disabled  SatFdbkVariant=Disabled  DerivativeFilterVariant=Disabled  NVariant=Disabled  NCopyVariant=Disabled_SignalSpec  FilterICVariant=Disabled  IntegratorICVariant=InternalICs  ExternalResetVariant=Disabled  TRSumVariant=Passthrough  SumFdbkVariant=Disabled  SumVariant=Sum_PI  TsampFilterVariant=InternalTs  TsampNgainVariant=Passthrough  TsampIntegralVariant=Passthrough  ExternalSaturationOutDataTypeStr=Inherit: Same as second input
  out_mod_x : Outport
  wires:
  Add/1 -> Data Type Conversion8/1
  actual_Mod_x/1 -> Add/2
  Data Type Conversion8/1 -> PID Controller2/1
  setp_Mod_x/1 -> Add/1
  PID Controller2/1 -> out_mod_x/1

== system uz_pmsm_model_9ph/Subsystem8/Subsystem3 ==
  setp_Mod_x : Inport
  actual_Mod_x : Inport  Port=2
  Add : Sum  Inputs=+-
  Data Type Conversion8 : DataTypeConversion  OutDataTypeStr=double
  PID Controller2 : slpidlib/PID Controller  Controller=PI  Form=Ideal  TimeDomain=Continuous-time  UseExternalTs=off  SampleTime=-1  IntegratorMethod=Forward Euler  FilterMethod=Forward Euler  ControllerParametersSource=internal  P=k_p_q  I=k_i_q  D=0  UseFilter=on  N=100  TunerSelectOption=Transfer Function Based (PID Tuner App)  InitialConditionSource=internal  InitialConditionForIntegrator=0  InitialConditionForFilter=0  DifferentiatorICPrevScaledInput=0  ExternalReset=none  TrackingMode=off  Kt=1  LimitOutput=on  SatLimitsSource=internal  UpperSaturationLimit=100  LowerSaturationLimit=-100  LinearizeAsGain=on  AntiWindupMode=clamping  Kb=1  POutMin=[]  POutMax=[]  IOutMin=[]  IOutMax=[]  DOutMin=[]  DOutMax=[]  NOutMin=[]  NOutMax=[]  SumOutMin=[]  SumOutMax=[]  SaturationOutMin=[]  SaturationOutMax=[]  PParamMin=[]  PParamMax=[]  IParamMin=[]  IParamMax=[]  DParamMin=[]  DParamMax=[]  NParamMin=[]  NParamMax=[]  KbParamMin=[]  KbParamMax=[]  KtParamMin=[]  KtParamMax=[]  KbOutMin=[]  KbOutMax=[]  KtOutMin=[]  KtOutMax=[]  IntegratorOutMin=[]  IntegratorOutMax=[]  FilterOutMin=[]  FilterOutMax=[]  SumI1OutMin=[]  SumI1OutMax=[]  SumI2OutMin=[]  SumI2OutMax=[]  SumI3OutMin=[]  SumI3OutMax=[]  SumI4OutMin=[]  SumI4OutMax=[]  SumDOutMin=[]  SumDOutMax=[]  DifferentiatorOutMin=[]  DifferentiatorOutMax=[]  FilterDiffOutCoefMin=[]  FilterDiffOutCoefMax=[]  ReciprocalOutMin=[]  ReciprocalOutMax=[]  SumDenOutMin=[]  SumDenOutMax=[]  SumNumOutMin=[]  SumNumOutMax=[]  DivideOutMin=[]  DivideOutMax=[]  UdiffTsProdOutMin=[]  UdiffTsProdOutMax=[]  NTsProdOutMin=[]  NTsProdOutMax=[]  UintegralTsProdOutMin=[]  UintegralTsProdOutMax=[]  UngainTsProdOutMin=[]  UngainTsProdOutMax=[]  IntegratorContinuousStateAttributes=''  IntegratorStateMustResolveToSignalObject=off  IntegratorRTWStateStorageClass=Auto  FilterContinuousStateAttributes=''  FilterStateMustResolveToSignalObject=off  FilterRTWStateStorageClass=Auto  ParallelPVariant=Passthrough  IdealPVariant=InternalParameters  IVariant=InternalParameters  DVariant=Disabled  IntegratorVariant=Continuous  SatVariant=Enabled  AWVariant=ContClampingIdeal  PCopyVariant=InternalParamsIdeal  TRVariant=Disabled  FdbkBlocksVariant=Forward  IdealPFdbkVariant=Disabled  SatFdbkVariant=Disabled  DerivativeFilterVariant=Disabled  NVariant=Disabled  NCopyVariant=Disabled_SignalSpec  FilterICVariant=Disabled  IntegratorICVariant=InternalICs  ExternalResetVariant=Disabled  TRSumVariant=Passthrough  SumFdbkVariant=Disabled  SumVariant=Sum_PI  TsampFilterVariant=InternalTs  TsampNgainVariant=Passthrough  TsampIntegralVariant=Passthrough  ExternalSaturationOutDataTypeStr=Inherit: Same as second input
  out_mod_x : Outport
  wires:
  PID Controller2/1 -> out_mod_x/1
  setp_Mod_x/1 -> Add/1
  Data Type Conversion8/1 -> PID Controller2/1
  actual_Mod_x/1 -> Add/2
  Add/1 -> Data Type Conversion8/1

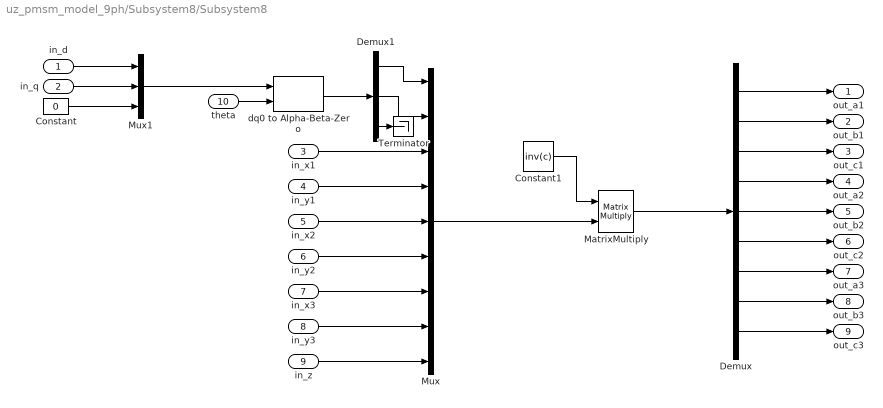
== system uz_pmsm_model_9ph/Subsystem8/Subsystem8 ==
  in_d : Inport
  in_q : Inport  Port=2
  in_x1 : Inport  Port=3
  in_y1 : Inport  Port=4
  in_x2 : Inport  Port=5
  in_y2 : Inport  Port=6
  in_x3 : Inport  Port=7
  in_y3 : Inport  Port=8
  in_z : Inport  Port=9
  theta : Inport  Port=10
  Constant : Constant  Value=0
  Constant1 : Constant  Value=inv(c)
  Demux : Demux  Outputs=9
  Demux1 : Demux  Outputs=3
  MatrixMultiply : Product  Multiplication=Matrix(*)
  Mux : Mux  Inputs=9
  Mux1 : Mux  Inputs=3
  Terminator : Terminator
  dq0 to Alpha-Beta-Zero : spsdq0toAlphaBetaZeroLib/dq0 to Alpha-Beta-Zero  Alignment=90 degrees behind phase A axis
      settings: SourceProductBaseCode=PS
  out_a1 : Outport
  out_b1 : Outport  Port=2
  out_c1 : Outport  Port=3
  out_a2 : Outport  Port=4
  out_b2 : Outport  Port=5
  out_c2 : Outport  Port=6
  out_a3 : Outport  Port=7
  out_b3 : Outport  Port=8
  out_c3 : Outport  Port=9
  wires:
  in_x3/1 -> Mux/7
  in_y3/1 -> Mux/8
  MatrixMultiply/1 -> Demux/1
  in_y2/1 -> Mux/6
  Demux/1 -> out_a1/1
  in_x1/1 -> Mux/3
  in_y1/1 -> Mux/4
  Mux/1 -> MatrixMultiply/2
  in_x2/1 -> Mux/5
  in_z/1 -> Mux/9
  Constant/1 -> Mux1/3
  in_q/1 -> Mux1/2
  in_d/1 -> Mux1/1
  Mux1/1 -> dq0 to Alpha-Beta-Zero/1
  theta/1 -> dq0 to Alpha-Beta-Zero/2
  dq0 to Alpha-Beta-Zero/1 -> Demux1/1
  Demux1/1 -> Mux/1
  Demux1/2 -> Mux/2
  Demux1/3 -> Terminator/1
  Constant1/1 -> MatrixMultiply/1
  Demux/2 -> out_b1/1
  Demux/3 -> out_c1/1
  Demux/4 -> out_a2/1
  Demux/6 -> out_c2/1
  Demux/5 -> out_b2/1
  Demux/8 -> out_b3/1
  Demux/9 -> out_c3/1
  Demux/7 -> out_a3/1

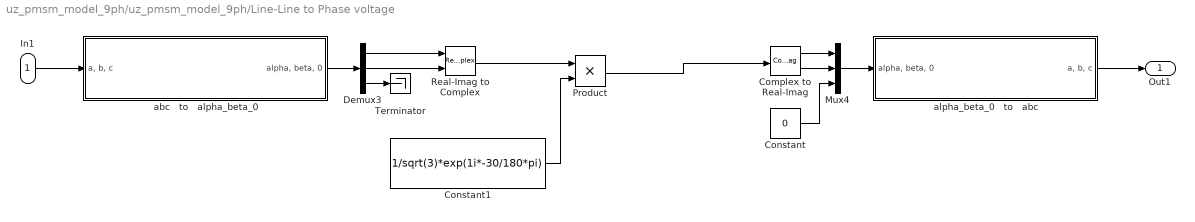
== system uz_pmsm_model_9ph/uz_pmsm_model_9ph/Line-Line to Phase voltage ==
  In1 : Inport
  Complex to Real-Imag : ComplexToRealImag
  Constant : Constant  Value=0  OutDataTypeStr=single  SampleTime=ts
  Constant1 : Constant  Value=1/sqrt(3)*exp(1i*-30/180*pi)  OutDataTypeStr=single  SampleTime=ts
  Demux3 : Demux  Outputs=3
  Mux4 : Mux  Inputs=3
  Product : Product  OutDataTypeStr=single
  Real-Imag to Complex : RealImagToComplex
  Terminator : Terminator
  abc   to   alpha_beta_0 : Subsystem
  alpha_beta_0   to   abc : Subsystem
  Out1 : Outport
  wires:
  Demux3/2 -> Real-Imag to Complex/2
  Complex to Real-Imag/1 -> Mux4/1
  Mux4/1 -> alpha_beta_0   to   abc/1("alpha, beta, 0  ")
  Product/1 -> Complex to Real-Imag/1
  Real-Imag to Complex/1 -> Product/1
  Demux3/1 -> Real-Imag to Complex/1
  Complex to Real-Imag/2 -> Mux4/2
  Constant/1 -> Mux4/3
  In1/1 -> abc   to   alpha_beta_0/1("a, b, c")
  Demux3/3 -> Terminator/1
  abc   to   alpha_beta_0/1("alpha, beta, 0 ") -> Demux3/1
  alpha_beta_0   to   abc/1("a, b, c") -> Out1/1
  Constant1/1 -> Product/2

== system uz_pmsm_model_9ph/uz_pmsm_model_9ph/Line-Line to Phase voltage1 ==
  In1 : Inport
  Complex to Real-Imag : ComplexToRealImag
  Constant : Constant  Value=0  OutDataTypeStr=single  SampleTime=ts
  Constant1 : Constant  Value=1/sqrt(3)*exp(1i*-30/180*pi)  OutDataTypeStr=single  SampleTime=ts
  Demux3 : Demux  Outputs=3
  Mux4 : Mux  Inputs=3
  Product : Product  OutDataTypeStr=single
  Real-Imag to Complex : RealImagToComplex
  Terminator : Terminator
  abc   to   alpha_beta_0 : Subsystem
  alpha_beta_0   to   abc : Subsystem
  Out1 : Outport
  wires:
  Constant1/1 -> Product/2
  alpha_beta_0   to   abc/1("a, b, c") -> Out1/1
  abc   to   alpha_beta_0/1("alpha, beta, 0 ") -> Demux3/1
  Demux3/3 -> Terminator/1
  In1/1 -> abc   to   alpha_beta_0/1("a, b, c")
  Constant/1 -> Mux4/3
  Complex to Real-Imag/2 -> Mux4/2
  Demux3/1 -> Real-Imag to Complex/1
  Real-Imag to Complex/1 -> Product/1
  Product/1 -> Complex to Real-Imag/1
  Mux4/1 -> alpha_beta_0   to   abc/1("alpha, beta, 0  ")
  Complex to Real-Imag/1 -> Mux4/1
  Demux3/2 -> Real-Imag to Complex/2

== system uz_pmsm_model_9ph/uz_pmsm_model_9ph/Line-Line to Phase voltage2 ==
  In1 : Inport
  Complex to Real-Imag : ComplexToRealImag
  Constant : Constant  Value=0  OutDataTypeStr=single  SampleTime=ts
  Constant1 : Constant  Value=1/sqrt(3)*exp(1i*-30/180*pi)  OutDataTypeStr=single  SampleTime=ts
  Demux3 : Demux  Outputs=3
  Mux4 : Mux  Inputs=3
  Product : Product  OutDataTypeStr=single
  Real-Imag to Complex : RealImagToComplex
  Terminator : Terminator
  abc   to   alpha_beta_0 : Subsystem
  alpha_beta_0   to   abc : Subsystem
  Out1 : Outport
  wires:
  Demux3/2 -> Real-Imag to Complex/2
  Complex to Real-Imag/1 -> Mux4/1
  Mux4/1 -> alpha_beta_0   to   abc/1("alpha, beta, 0  ")
  Product/1 -> Complex to Real-Imag/1
  Real-Imag to Complex/1 -> Product/1
  Demux3/1 -> Real-Imag to Complex/1
  Complex to Real-Imag/2 -> Mux4/2
  Constant/1 -> Mux4/3
  In1/1 -> abc   to   alpha_beta_0/1("a, b, c")
  Demux3/3 -> Terminator/1
  abc   to   alpha_beta_0/1("alpha, beta, 0 ") -> Demux3/1
  alpha_beta_0   to   abc/1("a, b, c") -> Out1/1
  Constant1/1 -> Product/2

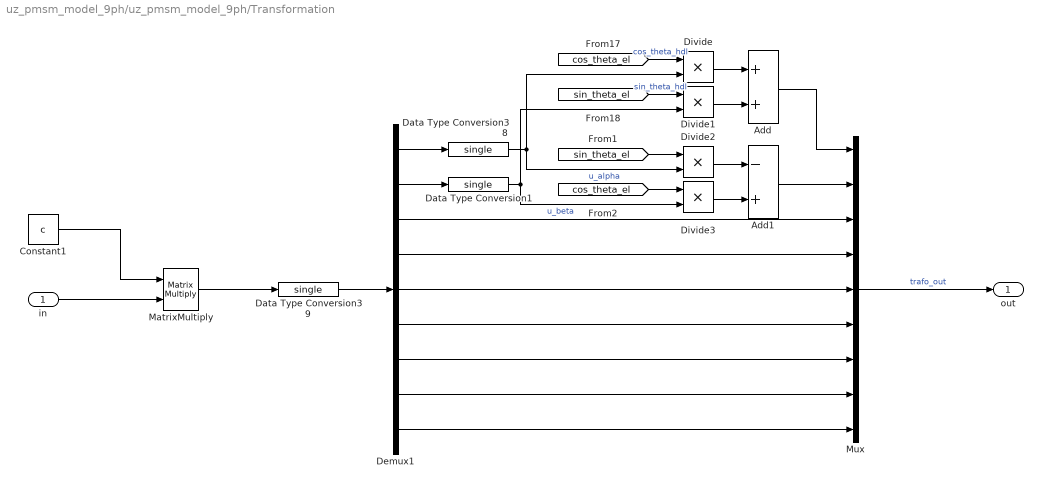
== system uz_pmsm_model_9ph/uz_pmsm_model_9ph/Transformation ==
  in : Inport
  Add : Sum
  Add1 : Sum  Inputs=-+
  Constant1 : Constant  Value=c  OutDataTypeStr=fixdt(1,18)  SampleTime=ts
  Data Type Conversion1 : DataTypeConversion  OutDataTypeStr=single  RndMeth=Nearest
  Data Type Conversion38 : DataTypeConversion  OutDataTypeStr=single  RndMeth=Nearest
  Data Type Conversion39 : DataTypeConversion  OutDataTypeStr=single  RndMeth=Nearest
  Demux1 : Demux  Outputs=9
  Divide{,1..3} (4 alike) : Product  Inputs=**
  MatrixMultiply : Product  Multiplication=Matrix(*)
  Mux : Mux  Inputs=9
  out : Outport
  wires:
  Demux1/3 -> Mux/3
  Demux1/4 -> Mux/4
  Demux1/5 -> Mux/5
  Demux1/6 -> Mux/6
  Demux1/7 -> Mux/7
  Demux1/8 -> Mux/8
  Demux1/9 -> Mux/9
  Mux/1 -> out/1  "trafo_out"
  Demux1/1 -> Data Type Conversion38/1
  Demux1/2 -> Data Type Conversion1/1
  Add1/1 -> Mux/2
  Add/1 -> Mux/1
  Data Type Conversion38/1 -> Divide/2, Divide2/2  "u_alpha"
  Data Type Conversion1/1 -> Divide1/2, Divide3/2  "u_beta"
  Divide/1 -> Add/1
  Divide1/1 -> Add/2
  [sin_theta_el] -> Divide1/1  "sin_theta_hdl"
  [cos_theta_el] -> Divide/1  "cos_theta_hdl"
  [sin_theta_el] -> Divide2/1
  [cos_theta_el] -> Divide3/1
  Divide3/1 -> Add1/2
  Divide2/1 -> Add1/1
  MatrixMultiply/1 -> Data Type Conversion39/1
  Constant1/1 -> MatrixMultiply/1
  Data Type Conversion39/1 -> Demux1/1
  in/1 -> MatrixMultiply/2

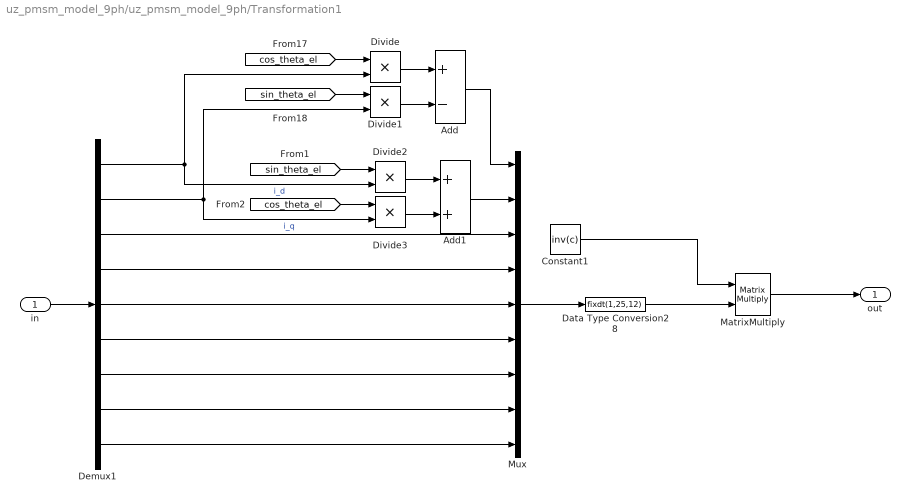
== system uz_pmsm_model_9ph/uz_pmsm_model_9ph/Transformation1 ==
  in : Inport
  Add : Sum  Inputs=+-
  Add1 : Sum
  Constant1 : Constant  Value=inv(c)  OutDataTypeStr=fixdt(1,18)  SampleTime=ts
  Data Type Conversion28 : DataTypeConversion  OutDataTypeStr=fixdt(1,25,12)  RndMeth=Nearest
  Demux1 : Demux  Outputs=9
  Divide{,1..3} (4 alike) : Product  Inputs=**
  MatrixMultiply : Product  Multiplication=Matrix(*)
  Mux : Mux  Inputs=9
  out : Outport
  wires:
  in/1 -> Demux1/1
  Mux/1 -> Data Type Conversion28/1
  Demux1/8 -> Mux/8
  Demux1/6 -> Mux/6
  Demux1/4 -> Mux/4
  Demux1/3 -> Mux/3
  Demux1/5 -> Mux/5
  Demux1/9 -> Mux/9
  Demux1/7 -> Mux/7
  [sin_theta_el] -> Divide1/1
  Demux1/2 -> Divide3/2, Divide1/2  "i_q"
  Add/1 -> Mux/1
  Divide/1 -> Add/1
  [cos_theta_el] -> Divide/1
  Divide1/1 -> Add/2
  Demux1/1 -> Divide2/2, Divide/2  "i_d"
  Divide3/1 -> Add1/2
  [sin_theta_el] -> Divide2/1
  Divide2/1 -> Add1/1
  [cos_theta_el] -> Divide3/1
  Add1/1 -> Mux/2
  Data Type Conversion28/1 -> MatrixMultiply/2
  Constant1/1 -> MatrixMultiply/1
  MatrixMultiply/1 -> out/1

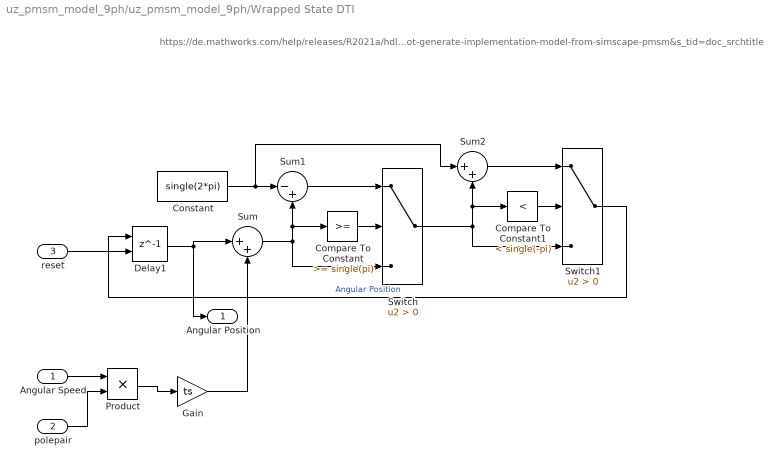
== system uz_pmsm_model_9ph/uz_pmsm_model_9ph/Wrapped State DTI ==
  note: https://de.mathworks.com/help/releases/R2021a/hdlcoder/ug/troubleshoot-generate-implementation-model-from-simscape-pmsm.html?searchHighlight=troubleshoot-generate-implementation-model-from-simscape-pmsm&s_tid=doc_srchtitle
  Angular Speed : Inport
  polepair : Inport  Port=2
  reset : Inport  Port=3
  Compare To Constant : simulink/Logic and Bit Operations/Compare To Constant  relop=>=  const=single(pi)  OutDataTypeStr=boolean
  Compare To Constant1 : simulink/Logic and Bit Operations/Compare To Constant  relop=<  const=single(-pi)  OutDataTypeStr=boolean
  Constant : Constant  Value=single(2*pi)  SampleTime=-1
  Delay1 : Delay  DelayLength=1  ExternalReset=Level
      settings: InputPortMap=u0,r5
  Gain : Gain  Gain=ts
  Product : Product
  Sum : Sum  Inputs=|++
  Sum1 : Sum  Inputs=|-+
  Sum2 : Sum  Inputs=|++
  Switch : Switch  Criteria=u2 > Threshold
  Switch1 : Switch  Criteria=u2 > Threshold
  Angular Position : Outport
  wires:
  Compare To Constant1/1 -> Switch1/2
  Delay1/1 -> Sum/1, Angular Position/1
  Constant/1 -> Sum2/1, Sum1/1
  Sum2/1 -> Switch1/1
  Switch1/1 -> Delay1/1  "Angular Position"
  Switch/1 -> Sum2/2, Compare To Constant1/1, Switch1/3
  Compare To Constant/1 -> Switch/2
  Sum/1 -> Compare To Constant/1, Sum1/2, Switch/3
  Sum1/1 -> Switch/1
  Gain/1 -> Sum/2
  reset/1 -> Delay1/2
  Product/1 -> Gain/1
  Angular Speed/1 -> Product/1
  polepair/1 -> Product/2

== system uz_pmsm_model_9ph/uz_pmsm_model_9ph/mechanical_system ==
  note: load torque negative!!!
  note: This delay breaks the algebraic loop between mechanical and electrical system.
      | Introduces a delay of 500ns.
  reset : Inport
  M_Mi : Inport  Port=2
  reciprocal_J : Inport  Port=3
  load_torque : Inport  Port=4
  Data Type Conversion1 : DataTypeConversion  OutDataTypeStr=double  RndMeth=Nearest
  Data Type Conversion8 : DataTypeConversion  OutDataTypeStr=single  RndMeth=Nearest
  Delay : Delay  DelayLength=1
  Product11 : Product
  Sum1 : Sum  Inputs=|++
  integrator : Subsystem
  omega_mech : Outport
  wires:
  Product11/1 -> Data Type Conversion1/1
  integrator/1(outt) -> Data Type Conversion8/1
  reciprocal_J/1 -> Product11/1
  Sum1/1 -> Product11/2
  load_torque/1 -> Sum1/2
  M_Mi/1 -> Delay/1
  Delay/1 -> Sum1/1
  Data Type Conversion8/1 -> omega_mech/1
  Data Type Conversion1/1 -> integrator/1(in)
  reset/1 -> integrator/2(reset)

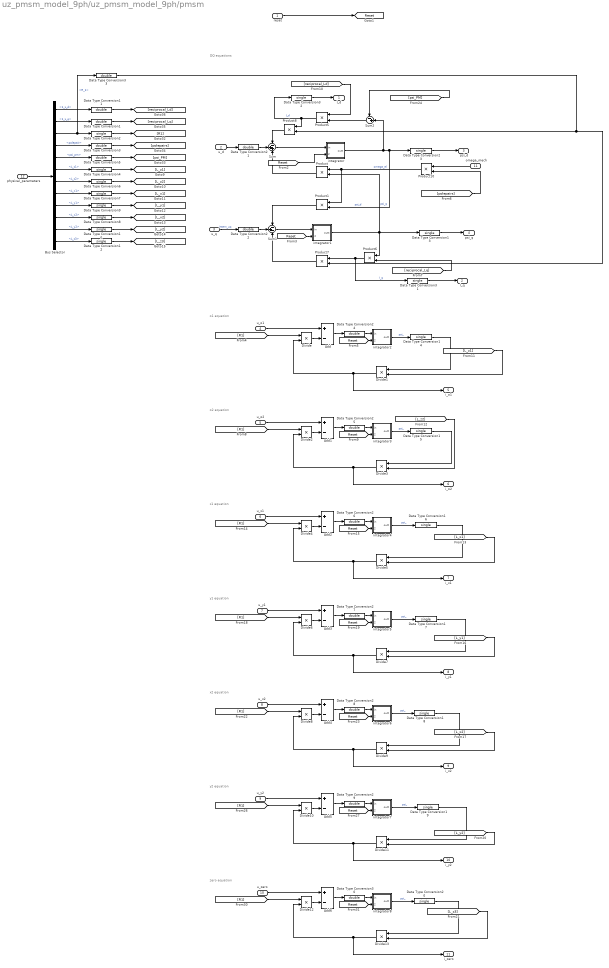
== system uz_pmsm_model_9ph/uz_pmsm_model_9ph/pmsm ==
  note: o1 equation
  note: DQ equations
  note: o2 equation
  note: x1 equation
  note: y1 equation
  note: x2 equation
  note: y2 equation
  note: zero equation
  reset : Inport
  u_d : Inport  Port=2
  u_q : Inport  Port=3
  u_o1 : Inport  Port=4
  u_o2 : Inport  Port=5
  u_x1 : Inport  Port=6
  u_y1 : Inport  Port=7
  u_x2 : Inport  Port=8
  u_y2 : Inport  Port=9
  u_zero : Inport  Port=10
  omega_mech : Inport  Port=11
  physical_parameters : Inport  Port=12
  Add{,1..6} (7 alike) : Sum  Inputs=+-
  Bus Selector : BusSelector  OutputSignals=1_L_d,1_L_q,R_1,polepair,psi_pm,L_z1,L_z2,L_x1,L_y1,L_x2,L_y2,L_z3
  Data Type Conversion{1,3,5,11,21..22,24..30,33} (14 alike) : DataTypeConversion  OutDataTypeStr=double  RndMeth=Nearest
  Data Type Conversion{2,4,6..10,12..20,23,31..32} (19 alike) : DataTypeConversion  OutDataTypeStr=single  RndMeth=Nearest
  Divide{,1..13} (14 alike) : Product  Inputs=**
  Product{,1,5..8,10} (7 alike) : Product
  Sum : Sum  Inputs=-++
  Sum1 : Sum  Inputs=-+-
  Sum2 : Sum  Inputs=-+|
  integrator : Subsystem
  integrator1 : Subsystem
  integrator2 : Subsystem
  integrator3 : Subsystem
  integrator4 : Subsystem
  integrator5 : Subsystem
  integrator6 : Subsystem
  integrator7 : Subsystem
  integrator8 : Subsystem
  I_d : Outport
  I_q : Outport  Port=2
  psi_d : Outport  Port=3
  psi_q : Outport  Port=4
  i_o1 : Outport  Port=5
  i_o2 : Outport  Port=6
  i_x1 : Outport  Port=7
  i_y1 : Outport  Port=8
  i_x2 : Outport  Port=9
  i_y2 : Outport  Port=10
  i_zero : Outport  Port=11
  tag scope: Reset=global
  wires:
  omega_mech/1 -> Product10/1
  u_q/1 -> Data Type Conversion22/1  "intern_uq"
  Product/1 -> Sum/3
  Product5/1 -> Data Type Conversion32/1, Product8/1  "I_d"
  [reciprocal_Ld] -> Product5/1
  integrator1/1(outt) -> Data Type Conversion13/1, Product/2, Product6/1  "psi_q"
  u_d/1 -> Data Type Conversion21/1
  Product1/1 -> Sum1/1
  [psi_PM] -> Sum2/1
  Product6/1 -> Data Type Conversion31/1, Product7/1  "I_q"
  Product10/1 -> Product1/1, Product/1  "omega_el"
  integrator/1(outt) -> Sum2/2, Product1/2, Data Type Conversion23/1  "psi_d"
  Sum2/1 -> Product5/2
  Product8/1 -> Sum/1
  [reciprocal_Lq] -> Product6/2
  Product7/1 -> Sum1/3
  Data Type Conversion33/1 -> Product8/2, Product7/2
  reset/1 -> [Reset]
  [Reset] -> integrator/2(reset)
  [Reset] -> integrator1/2(reset)
  [Reset] -> integrator2/2(reset)
  [L_z1] -> Divide1/2
  u_o1/1 -> Add/1
  Divide1/1 -> i_o1/1, Divide/2
  Divide/1 -> Add/2
  Add/1 -> Data Type Conversion24/1
  [R1] -> Divide/1
  integrator2/1(outt) -> Data Type Conversion14/1  "psi_"
  integrator3/1(outt) -> Data Type Conversion15/1  "psi_"
  [R1] -> Divide2/1
  Add1/1 -> Data Type Conversion25/1
  Divide2/1 -> Add1/2
  Divide3/1 -> i_o2/1, Divide2/2
  u_o2/1 -> Add1/1
  [L_z2] -> Divide3/2
  [Reset] -> integrator3/2(reset)
  [Reset] -> integrator4/2(reset)
  u_x1/1 -> Add2/1
  Divide5/1 -> i_x1/1, Divide4/2
  Divide4/1 -> Add2/2
  Add2/1 -> Data Type Conversion26/1
  [R1] -> Divide4/1
  integrator4/1(outt) -> Data Type Conversion16/1  "psi_"
  integrator5/1(outt) -> Data Type Conversion17/1  "psi_"
  [R1] -> Divide6/1
  Add3/1 -> Data Type Conversion27/1
  Divide6/1 -> Add3/2
  Divide7/1 -> i_y1/1, Divide6/2
  u_y1/1 -> Add3/1
  [Reset] -> integrator5/2(reset)
  [Reset] -> integrator6/2(reset)
  u_x2/1 -> Add4/1
  Divide9/1 -> i_x2/1, Divide8/2
  Divide8/1 -> Add4/2
  Add4/1 -> Data Type Conversion28/1
  [R1] -> Divide8/1
  integrator6/1(outt) -> Data Type Conversion18/1  "psi_"
  integrator7/1(outt) -> Data Type Conversion19/1  "psi_"
  [R1] -> Divide10/1
  Add5/1 -> Data Type Conversion29/1
  Divide10/1 -> Add5/2
  Divide11/1 -> i_y2/1, Divide10/2
  u_y2/1 -> Add5/1
  [Reset] -> integrator7/2(reset)
  [Reset] -> integrator8/2(reset)
  u_zero/1 -> Add6/1
  Divide13/1 -> i_zero/1, Divide12/2
  Divide12/1 -> Add6/2
  Add6/1 -> Data Type Conversion30/1
  [R1] -> Divide12/1
  integrator8/1(outt) -> Data Type Conversion20/1  "psi_"
  Bus Selector/1 -> Data Type Conversion11/1  "<1_L_d>"
  Data Type Conversion12/1 -> [L_z3]
  Data Type Conversion9/1 -> [L_y1]
  Data Type Conversion1/1 -> [reciprocal_Lq]
  Data Type Conversion5/1 -> [psi_PM]
  Bus Selector/4 -> Data Type Conversion3/1  "<polepair>"
  Bus Selector/8 -> Data Type Conversion7/1  "<L_x1>"
  Bus Selector/2 -> Data Type Conversion1/1  "<1_L_q>"
  Bus Selector/5 -> Data Type Conversion5/1  "<psi_pm>"
  Data Type Conversion8/1 -> [L_x2]
  Data Type Conversion10/1 -> [L_y2]
  Bus Selector/6 -> Data Type Conversion4/1  "<L_z1>"
  Bus Selector/7 -> Data Type Conversion6/1  "<L_z2>"
  Data Type Conversion7/1 -> [L_x1]
  Data Type Conversion6/1 -> [L_z2]
  Bus Selector/11 -> Data Type Conversion10/1  "<L_y2>"
  Bus Selector/12 -> Data Type Conversion12/1  "<L_z3>"
  Bus Selector/3 -> Data Type Conversion33/1, Data Type Conversion2/1  "<R_1>"
  Bus Selector/10 -> Data Type Conversion8/1  "<L_x2>"
  Data Type Conversion4/1 -> [L_z1]
  physical_parameters/1 -> Bus Selector/1
  Data Type Conversion3/1 -> [polepairs]
  Data Type Conversion11/1 -> [reciprocal_Ld]
  Bus Selector/9 -> Data Type Conversion9/1  "<L_y1>"
  Data Type Conversion2/1 -> [R1]
  [polepairs] -> Product10/2
  [L_x1] -> Divide5/2
  [L_y1] -> Divide7/2
  [L_x2] -> Divide9/2
  [L_y2] -> Divide11/2
  [L_z3] -> Divide13/2
  Data Type Conversion14/1 -> Divide1/1
  Data Type Conversion15/1 -> Divide3/1
  Data Type Conversion16/1 -> Divide5/1
  Data Type Conversion17/1 -> Divide7/1
  Data Type Conversion18/1 -> Divide9/1
  Data Type Conversion19/1 -> Divide11/1
  Data Type Conversion20/1 -> Divide13/1
  Sum/1 -> integrator/1(in)
  Sum1/1 -> integrator1/1(in)
  Data Type Conversion24/1 -> integrator2/1(in)
  Data Type Conversion25/1 -> integrator3/1(in)
  Data Type Conversion26/1 -> integrator4/1(in)
  Data Type Conversion27/1 -> integrator5/1(in)
  Data Type Conversion28/1 -> integrator6/1(in)
  Data Type Conversion29/1 -> integrator7/1(in)
  Data Type Conversion30/1 -> integrator8/1(in)
  Data Type Conversion22/1 -> Sum1/2
  Data Type Conversion13/1 -> psi_q/1
  Data Type Conversion31/1 -> I_q/1
  Data Type Conversion21/1 -> Sum/2
  Data Type Conversion23/1 -> psi_d/1
  Data Type Conversion32/1 -> I_d/1

== system uz_pmsm_model_9ph/uz_pmsm_model_9ph/torque_calculation ==
  I_d : Inport
  I_q : Inport  Port=2
  psi_d : Inport  Port=3
  psi_q : Inport  Port=4
  polepairs : Inport  Port=5
  Factor : Gain  Gain=9/2
  Product2 : Product
  Product3 : Product
  Product9 : Product
  Sum3 : Sum  Inputs=-|+
  M_Mi : Outport
  wires:
  Sum3/1 -> Factor/1
  Product3/1 -> Sum3/2
  Product2/1 -> Sum3/1
  psi_q/1 -> Product2/2
  psi_d/1 -> Product3/1
  I_d/1 -> Product2/1
  I_q/1 -> Product3/2
  Product9/1 -> M_Mi/1  "M_Mi"
  polepairs/1 -> Product9/2
  Factor/1 -> Product9/1  "M_Mi"

== system uz_pmsm_model_9ph/uz_pmsm_model_9ph/Line-Line to Phase voltage/abc   to   alpha_beta_0 ==
  "a, b, c" : Inport  PortDimensions=3
  Gain2 : Gain  Gain=2/3  SaturateOnIntegerOverflow=on  OutDataTypeStr=Inherit: Same as input  ParamDataTypeStr=Inherit: Same as input
  Gain4 : Gain  Gain="[ 1   -0.5   -0.5; 0   0.5*sqrt(3)   -0.5*sqrt(3); 0.5  0.5  0.5 ]"  Multiplication=Matrix(K*u) (u vector)  SaturateOnIntegerOverflow=on  OutDataTypeStr=Inherit: Same as input  ParamDataTypeStr=Inherit: Same as input
  "alpha, beta, 0 " : Outport
  wires:
  Gain2/1 -> "alpha, beta, 0 "/1
  "a, b, c"/1 -> Gain4/1
  Gain4/1 -> Gain2/1

== system uz_pmsm_model_9ph/uz_pmsm_model_9ph/Line-Line to Phase voltage/alpha_beta_0   to   abc ==
  "alpha, beta, 0  " : Inport  PortDimensions=3
  Gain4 : Gain  Gain="[ 1 0 1; -0.5   0.5*sqrt(3)  1; -0.5 -0.5*sqrt(3) 1 ]"  Multiplication=Matrix(K*u) (u vector)  SaturateOnIntegerOverflow=on  OutDataTypeStr=Inherit: Same as input  ParamDataTypeStr=Inherit: Same as input
  "a, b, c" : Outport
  wires:
  Gain4/1 -> "a, b, c"/1
  "alpha, beta, 0  "/1 -> Gain4/1
